simulink subsystem "QuaternionInit"  (R2021a)
settings: Solver=VariableStepAuto  StartTime=0.0  StopTime=10.0  RelTol=1e-3
undefined symbols (not defined in the file): config
libraries: attitude_library x1
settings Model: Creator=Laura  LastModifiedBy=Laura

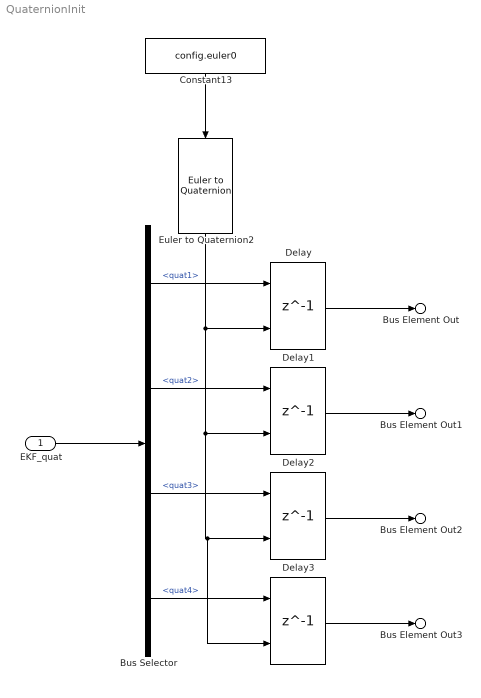
== system QuaternionInit ==
  EKF_quat : Inport
  Bus Selector : BusSelector  OutputSignals=quat1,quat2,quat3,quat4
  Constant13 : Constant  Value=config.euler0
  Delay{,1..3} (4 alike) : Delay  DelayLength=1  InitialConditionSource=Input port
      settings: InputPortMap=u0,p4
  Euler to Quaternion2 : attitude_library/Euler to Quaternion  SystemSampleTime=-1  VariantActivationTime=update diagram  Latency=0  AutoFrameSizeCalculation=off
      settings: SourceProductName=Attitude library
  Bus Element Out : Outport  PortName=EKF_quatbefore  Element=quat1
  Bus Element Out1 : Outport  PortName=EKF_quatbefore  Element=quat2
  Bus Element Out2 : Outport  PortName=EKF_quatbefore  Element=quat3
  Bus Element Out3 : Outport  PortName=EKF_quatbefore  Element=quat4
  wires:
  Euler to Quaternion2/1 -> Delay3/2, Delay2/2, Delay1/2, Delay/2
  Delay/1 -> Bus Element Out/1
  Delay1/1 -> Bus Element Out1/1
  Delay2/1 -> Bus Element Out2/1
  Delay3/1 -> Bus Element Out3/1
  EKF_quat/1 -> Bus Selector/1
  Bus Selector/1 -> Delay/1  "<quat1>"
  Bus Selector/2 -> Delay1/1  "<quat2>"
  Bus Selector/3 -> Delay2/1  "<quat3>"
  Bus Selector/4 -> Delay3/1  "<quat4>"
  Constant13/1 -> Euler to Quaternion2/1
